simulink model "logging"  (R2021b)
settings: Solver=VariableStepAuto  StartTime=0.0  StopTime=10.0  RelTol=1e-3
undefined symbols (not defined in the file): DiscIntNeverNeededParam, magnitude, Newton, Raphson
libraries: simulink x4, slpidlib x1
settings Model: Creator=user  LastModifiedBy=cemery

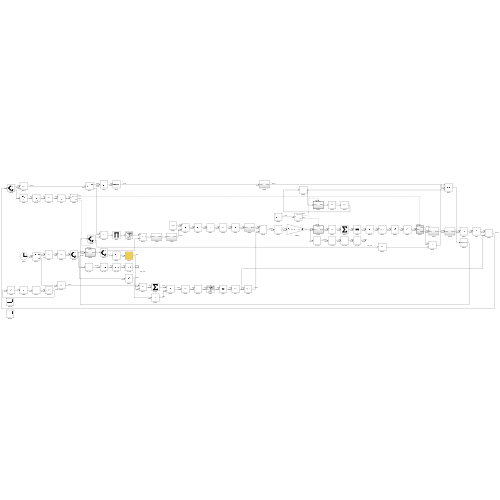
[thumbnail: Simulink's stored preview of the top-level diagram]
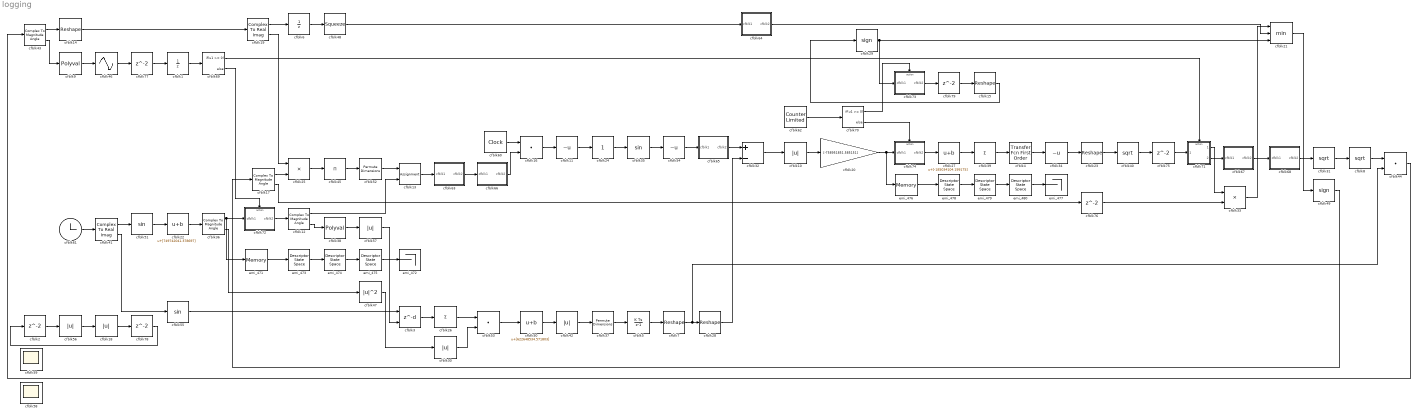
== system logging ==
  cfblk1 : UnitDelay  HasFrameUpgradeWarning=on
  cfblk{10,18,30,42,56..57} (6 alike) : Abs
  cfblk11 : UnaryMinus
  cfblk{12,17,36,43} (4 alike) : ComplexToMagnitudeAngle
  cfblk13 : Assignment  DiagnosticForDimensions=Warning  IndexOptions=Index vector (dialog)  Indices=1  OutputSizes=1
  cfblk{7,14..15,23,28} (5 alike) : Reshape
  cfblk16 : DotProduct  InputSameDT=on  OutDataTypeStr=Inherit: Inherit via internal rule
  cfblk19 : ComplexToRealImag
  cfblk{2,75..79} (6 alike) : Delay  SampleTime=1
  cfblk20 : Gain  Gain=[-758951851.585151]
  cfblk21 : MinMax  Inputs=3
  cfblk22 : Bias  Bias=[749742041.378697]
  cfblk24 : simulink/Math Operations/Slider Gain  gain=1  low=0  high=2
  cfblk25 : Product
  cfblk26 : Sum  Inputs=+
  cfblk27 : Bias  Bias=[-185034104.199175]
  cfblk29 : Signum
  cfblk3 : Delay  DelayLengthSource=Input port  SampleTime=1
      settings: InputPortMap=u0,p1
  cfblk31 : Sqrt  SaturateOnIntegerOverflow=on
  cfblk32 : Sum  Inputs=+-
  cfblk33 : Product
  cfblk34 : UnaryMinus
  cfblk35 : Trigonometry
  cfblk37 : PermuteDimensions
  cfblk38 : Polyval  Coefs=[ +2.081618890e-019, -1.441693666e-014, +4.719686976e-010, -8.536869453e-006, +1.621573104e-001, -8.087801117e+001 ]
  cfblk39 : Sum  Inputs=+
  cfblk4 : simulink/Discrete/Transfer Fcn First Order  PoleZ=0.95  ICPrevOutput=0.0  DoSatur=off
  cfblk40 : Sqrt  SaturateOnIntegerOverflow=on
  cfblk41 : ComplexToRealImag
  cfblk44 : DotProduct  InputSameDT=on  OutDataTypeStr=Inherit: Inherit via internal rule
  cfblk45 : Product  Inputs=*
  cfblk46 : Sin  TimeSource=Use external signal  SampleTime=0
  cfblk47 : Math  Operator=magnitude^2  SaturateOnIntegerOverflow=on
  cfblk48 : Squeeze
  cfblk49 : Signum
  cfblk5 : DiscreteIntegrator  ICPrevOutput=DiscIntNeverNeededParam  ICPrevScaledInput=DiscIntNeverNeededParam
  cfblk50 : Bias  Bias=[622648534.571803]
  cfblk51 : Trigonometry
  cfblk52 : PermuteDimensions
  cfblk53 : DotProduct  InputSameDT=on  OutDataTypeStr=Inherit: Inherit via internal rule
  cfblk54 : UnaryMinus
  cfblk55 : Trigonometry
  cfblk58 : Scope
      settings: Floating=on
  cfblk59 : Scope
      settings: Floating=on
  cfblk6 : UnitDelay  HasFrameUpgradeWarning=on
  cfblk60 : DigitalClock
  cfblk61 : Clock
  cfblk62 : simulink/Sources/Counter Limited  uplimit=[209.000000]  tsamp=-1
  cfblk63 : Subsystem
  cfblk64 : Subsystem
  cfblk65 : Subsystem
  cfblk66 : Subsystem
  cfblk67 : Subsystem
  cfblk68 : Subsystem
  cfblk69 : If  IfExpression=u1 >= 0  SampleTime=1
  cfblk70 : If  IfExpression=u1 >= 0  SampleTime=1
  cfblk71 : Subsystem  TreatAsAtomicUnit=on
  cfblk72 : Subsystem  TreatAsAtomicUnit=on
  cfblk73 : Subsystem  TreatAsAtomicUnit=on
  cfblk74 : Subsystem  TreatAsAtomicUnit=on
  cfblk8 : Sqrt  SaturateOnIntegerOverflow=on
  cfblk9 : Polyval  Coefs=[ +2.081618890e-019, -1.441693666e-014, +4.719686976e-010, -8.536869453e-006, +1.621573104e-001, -8.087801117e+001 ]
  emi_471 : Memory
  emi_472 : Terminator
  emi_{473..475,478..480} (6 alike) : DescriptorStateSpace
  emi_476 : Memory
  emi_477 : Terminator
  wires:
  cfblk47/1 -> cfblk30/1
  cfblk12/2 -> cfblk38/1
  emi_473/1 -> emi_474/1
  cfblk74/1(cfblk2) -> cfblk27/1
  cfblk18/1 -> cfblk78/1
  emi_480/1 -> emi_477/1
  emi_474/1 -> emi_475/1
  cfblk71/2(cfblk4) -> cfblk67/1(cfblk1)
  emi_479/1 -> emi_480/1
  cfblk68/1(cfblk2) -> cfblk31/1
  emi_478/1 -> emi_479/1
  cfblk78/1 -> cfblk2/1
  emi_476/1 -> emi_478/1
  cfblk77/1 -> cfblk1/1
  cfblk72/1(cfblk2) -> cfblk12/1
  cfblk66/1(cfblk2) -> cfblk16/2
  emi_475/1 -> emi_472/1
  emi_471/1 -> emi_473/1
  cfblk69/2 -> cfblk72/Action
  cfblk79/1 -> cfblk15/1
  cfblk62/1 -> cfblk70/1
  cfblk73/1(cfblk2) -> cfblk79/1
  cfblk19/2 -> cfblk25/1
  cfblk55/1 -> cfblk3/1
  cfblk76/1 -> cfblk33/2
  cfblk46/1 -> cfblk77/1
  cfblk54/1 -> cfblk65/1(cfblk1)
  cfblk17/2 -> cfblk76/1
  cfblk19/1 -> cfblk6/1
  cfblk75/1 -> cfblk71/1(cfblk1)
  cfblk21/1 -> cfblk49/1
  cfblk6/1 -> cfblk48/1
  cfblk70/2 -> cfblk74/Action
  cfblk40/1 -> cfblk75/1
  cfblk69/1 -> cfblk71/Action
  cfblk70/1 -> cfblk73/Action
  cfblk41/1 -> cfblk51/1
  cfblk67/1(cfblk2) -> cfblk68/1(cfblk1)
  cfblk28/1 -> cfblk32/2
  cfblk51/1 -> cfblk22/1
  cfblk61/1 -> cfblk41/1
  cfblk17/1 -> cfblk25/2
  cfblk52/1 -> cfblk13/1
  cfblk49/1 -> cfblk17/1
  cfblk10/1 -> cfblk20/1
  cfblk1/1 -> cfblk69/1
  cfblk3/1 -> cfblk26/1
  cfblk57/1 -> cfblk3/2
  cfblk2/1 -> cfblk56/1
  cfblk71/1(cfblk2) -> cfblk33/1
  cfblk50/1 -> cfblk42/1
  cfblk30/1 -> cfblk53/2
  cfblk14/1 -> cfblk19/1
  cfblk37/1 -> cfblk5/1
  cfblk41/2 -> cfblk55/1
  cfblk36/2 -> cfblk47/1
  cfblk64/1(cfblk2) -> cfblk21/2
  cfblk12/1 -> cfblk13/2
  cfblk53/1 -> cfblk50/1
  cfblk33/1 -> cfblk21/1
  cfblk16/1 -> cfblk11/1
  cfblk25/1 -> cfblk45/1
  cfblk60/1 -> cfblk16/1
  cfblk45/1 -> cfblk52/1
  cfblk15/1 -> cfblk29/1
  cfblk38/1 -> cfblk57/1
  cfblk9/1 -> cfblk46/1
  cfblk27/1 -> cfblk39/1
  cfblk32/1 -> cfblk10/1
  cfblk11/1 -> cfblk24/1
  cfblk22/1 -> cfblk36/1
  cfblk26/1 -> cfblk53/1
  cfblk44/1 -> cfblk43/1
  cfblk34/1 -> cfblk23/1
  cfblk8/1 -> cfblk44/1
  cfblk63/1(cfblk2) -> cfblk66/1(cfblk1)
  cfblk48/1 -> cfblk64/1(cfblk1)
  cfblk65/1(cfblk2) -> cfblk32/1
  cfblk31/1 -> cfblk8/1
  cfblk35/1 -> cfblk54/1
  cfblk4/1 -> cfblk34/1
  cfblk24/1 -> cfblk35/1
  cfblk43/2 -> cfblk9/1
  cfblk23/1 -> cfblk40/1
  cfblk13/1 -> cfblk63/1(cfblk1)
  cfblk42/1 -> cfblk37/1
  cfblk39/1 -> cfblk4/1
  cfblk43/1 -> cfblk14/1
  cfblk56/1 -> cfblk18/1
  cfblk5/1 -> cfblk7/1
  cfblk20/1 -> emi_476/1, cfblk74/1(cfblk1)
  cfblk36/1 -> emi_471/1, cfblk72/1(cfblk1)
  cfblk7/1 -> cfblk28/1, cfblk44/2
  cfblk29/1 -> cfblk73/1(cfblk1), cfblk21/3

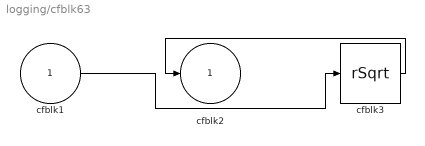
== system logging/cfblk63 ==
  cfblk1 : Inport
  cfblk3 : Sqrt  Operator=rSqrt  AlgorithmType=Newton-Raphson  SaturateOnIntegerOverflow=on
  cfblk2 : Outport
  wires:
  cfblk3/1 -> cfblk2/1
  cfblk1/1 -> cfblk3/1

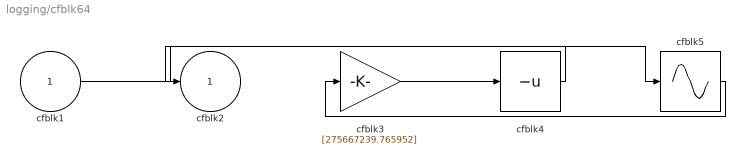
== system logging/cfblk64 ==
  cfblk1 : Inport
  cfblk3 : Gain  Gain=[275667239.765952]
  cfblk4 : UnaryMinus
  cfblk5 : Sin  TimeSource=Use external signal  SampleTime=0
  cfblk2 : Outport
  wires:
  cfblk1/1 -> cfblk5/1
  cfblk3/1 -> cfblk4/1
  cfblk5/1 -> cfblk3/1
  cfblk4/1 -> cfblk2/1

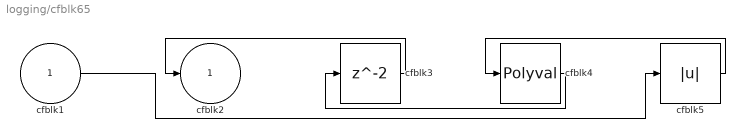
== system logging/cfblk65 ==
  cfblk1 : Inport
  cfblk3 : Delay  SampleTime=1
  cfblk4 : Polyval  Coefs=[ +2.081618890e-019, -1.441693666e-014, +4.719686976e-010, -8.536869453e-006, +1.621573104e-001, -8.087801117e+001 ]
  cfblk5 : Abs
  cfblk2 : Outport
  wires:
  cfblk3/1 -> cfblk2/1
  cfblk5/1 -> cfblk4/1
  cfblk4/1 -> cfblk3/1
  cfblk1/1 -> cfblk5/1

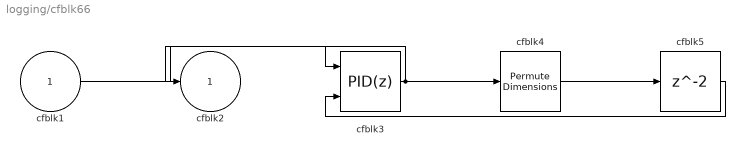
== system logging/cfblk66 ==
  cfblk1 : Inport
  cfblk3 : slpidlib/PID Controller (2DOF)  Controller=PID  Form=Parallel  TimeDomain=Discrete-time  UseExternalTs=off  SampleTime=1  IntegratorMethod=Forward Euler  FilterMethod=Forward Euler  ControllerParametersSource=internal  P=1  I=1  D=0  UseFilter=on  N=100  b=1  c=1  TunerSelectOption=Transfer Function Based (PID Tuner App)  InitialConditionSource=internal  InitialConditionForIntegrator=0  InitialConditionForFilter=0  DifferentiatorICPrevScaledInput=0  ExternalReset=none  TrackingMode=off  Kt=1  LimitOutput=off  SatLimitsSource=internal  UpperSaturationLimit=inf  LowerSaturationLimit=-inf  LinearizeAsGain=off  AntiWindupMode=none  Kb=1  POutMin=[]  POutMax=[]  IOutMin=[]  IOutMax=[]  DOutMin=[]  DOutMax=[]  NOutMin=[]  NOutMax=[]  bOutMin=[]  bOutMax=[]  cOutMin=[]  cOutMax=[]  SumOutMin=[]  SumOutMax=[]  SaturationOutMin=[]  SaturationOutMax=[]  PParamMin=[]  PParamMax=[]  IParamMin=[]  IParamMax=[]  DParamMin=[]  DParamMax=[]  NParamMin=[]  NParamMax=[]  bParamMin=[]  bParamMax=[]  cParamMin=[]  cParamMax=[]  KbParamMin=[]  KbParamMax=[]  KtParamMin=[]  KtParamMax=[]  KbOutMin=[]  KbOutMax=[]  KtOutMin=[]  KtOutMax=[]  IntegratorOutMin=[]  IntegratorOutMax=[]  FilterOutMin=[]  FilterOutMax=[]  SumI1OutMin=[]  SumI1OutMax=[]  SumI2OutMin=[]  SumI2OutMax=[]  SumI3OutMin=[]  SumI3OutMax=[]  SumI4OutMin=[]  SumI4OutMax=[]  SumDOutMin=[]  SumDOutMax=[]  Sum1OutMin=[]  Sum1OutMax=[]  Sum2OutMin=[]  Sum2OutMax=[]  Sum3OutMin=[]  Sum3OutMax=[]  DifferentiatorOutMin=[]  DifferentiatorOutMax=[]  FilterDiffOutCoefMin=[]  FilterDiffOutCoefMax=[]  ReciprocalOutMin=[]  ReciprocalOutMax=[]  SumDenOutMin=[]  SumDenOutMax=[]  SumNumOutMin=[]  SumNumOutMax=[]  DivideOutMin=[]  DivideOutMax=[]  UdiffTsProdOutMin=[]  UdiffTsProdOutMax=[]  NTsProdOutMin=[]  NTsProdOutMax=[]  UintegralTsProdOutMin=[]  UintegralTsProdOutMax=[]  UngainTsProdOutMin=[]  UngainTsProdOutMax=[]  IntegratorContinuousStateAttributes=''  IntegratorStateMustResolveToSignalObject=off  IntegratorRTWStateStorageClass=Auto  FilterContinuousStateAttributes=''  FilterStateMustResolveToSignalObject=off  FilterRTWStateStorageClass=Auto  ParallelPVariant=InternalParameters  IdealPVariant=Disabled  IVariant=InternalParameters  DVariant=InternalParameters  bVariant=InternalParameters  cVariant=InternalParameters  IntegratorVariant=Discrete  SatVariant=Disabled  AWVariant=Passthrough  PCopyVariant=Disabled  TRVariant=Disabled  FdbkBlocksVariant=Forward  IdealPFdbkVariant=Disabled  SatFdbkVariant=Disabled  DerivativeFilterVariant=ForwardEulerFilter  NVariant=InternalParameters  NCopyVariant=Disabled  FilterICVariant=InternalICsFilter  IntegratorICVariant=InternalICs  ExternalResetVariant=Disabled  TRSumVariant=Passthrough  SumFdbkVariant=Disabled  SumVariant=Sum_PID  TsampFilterVariant=InternalTs  TsampNgainVariant=Passthrough  TsampIntegralVariant=Passthrough  ExternalSaturationOutDataTypeStr=Inherit: Same as second input
      settings: SourceProductBaseCode=SL
  cfblk4 : PermuteDimensions
  cfblk5 : Delay  SampleTime=1
  cfblk2 : Outport
  wires:
  cfblk3/1 -> cfblk4/1, cfblk2/1
  cfblk1/1 -> cfblk3/1
  cfblk4/1 -> cfblk5/1
  cfblk5/1 -> cfblk3/2

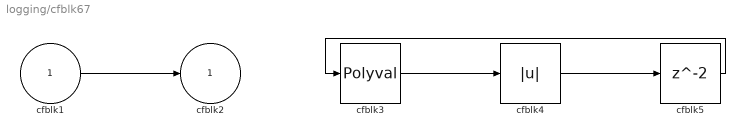
== system logging/cfblk67 ==
  cfblk1 : Inport
  cfblk3 : Polyval  Coefs=[ +2.081618890e-019, -1.441693666e-014, +4.719686976e-010, -8.536869453e-006, +1.621573104e-001, -8.087801117e+001 ]
  cfblk4 : Abs
  cfblk5 : Delay  SampleTime=1
  cfblk2 : Outport
  wires:
  cfblk1/1 -> cfblk2/1
  cfblk3/1 -> cfblk4/1
  cfblk4/1 -> cfblk5/1
  cfblk5/1 -> cfblk3/1

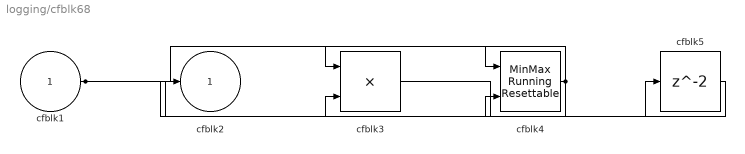
== system logging/cfblk68 ==
  cfblk1 : Inport
  cfblk3 : Product
  cfblk4 : simulink/Math Operations/MinMax Running Resettable  Function=min  vinit=0.0
  cfblk5 : Delay  SampleTime=1
  cfblk2 : Outport
  wires:
  cfblk1/1 -> cfblk4/1, cfblk3/2
  cfblk4/1 -> cfblk2/1, cfblk3/1
  cfblk3/1 -> cfblk5/1
  cfblk5/1 -> cfblk4/2

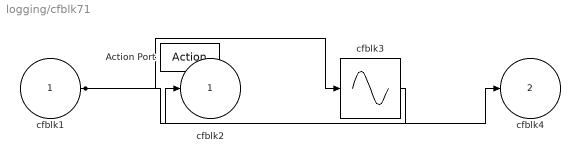
== system logging/cfblk71 ==
  cfblk1 : Inport
  Action Port : ActionPort  ActionPortLabel=if(u1 >= 0)
  cfblk3 : Sin  TimeSource=Use external signal  SampleTime=0
  cfblk2 : Outport
  cfblk4 : Outport  Port=2
  wires:
  cfblk3/1 -> cfblk2/1
  cfblk1/1 -> cfblk3/1, cfblk4/1

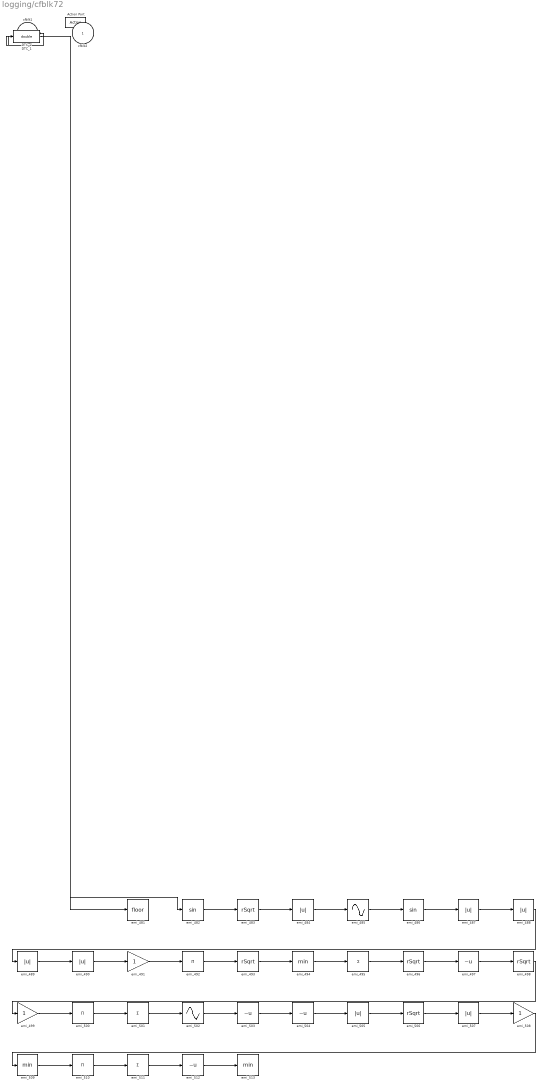
== system logging/cfblk72 ==
  cfblk1 : Inport
  Action Port : ActionPort  ActionPortLabel=else
  DTC_1 : DataTypeConversion  OutDataTypeStr=double
  DTC_2 : DataTypeConversion  OutDataTypeStr=double
  emi_481 : Rounding
  emi_482 : Trigonometry
  emi_{483,493,496,498,506} (5 alike) : Sqrt  Operator=rSqrt  SaturateOnIntegerOverflow=on
  emi_{484,487..490,505,507} (7 alike) : Abs
  emi_485 : Sin  TimeSource=Use external signal  SampleTime=0
  emi_486 : Trigonometry
  emi_491 : Gain
  emi_492 : Product  Inputs=*
  emi_494 : MinMax
  emi_495 : Sum  Inputs=+
  emi_{497,503..504,512} (4 alike) : UnaryMinus
  emi_499 : Gain
  emi_500 : Product  Inputs=*
  emi_501 : Sum  Inputs=+
  emi_502 : Sin  TimeSource=Use external signal  SampleTime=0
  emi_508 : Gain
  emi_509 : MinMax
  emi_510 : Product  Inputs=*
  emi_511 : Sum  Inputs=+
  emi_513 : MinMax
  cfblk2 : Outport
  wires:
  cfblk1/1 -> DTC_1/1, DTC_2/1
  DTC_1/1 -> emi_481/1
  DTC_2/1 -> emi_482/1
  emi_482/1 -> emi_483/1
  emi_483/1 -> emi_484/1
  emi_484/1 -> emi_485/1
  emi_485/1 -> emi_486/1
  emi_486/1 -> emi_487/1
  emi_487/1 -> emi_488/1
  emi_488/1 -> emi_489/1
  emi_489/1 -> emi_490/1
  emi_490/1 -> emi_491/1
  emi_491/1 -> emi_492/1
  emi_492/1 -> emi_493/1
  emi_493/1 -> emi_494/1
  emi_494/1 -> emi_495/1
  emi_495/1 -> emi_496/1
  emi_496/1 -> emi_497/1
  emi_497/1 -> emi_498/1
  emi_498/1 -> emi_499/1
  emi_499/1 -> emi_500/1
  emi_500/1 -> emi_501/1
  emi_501/1 -> emi_502/1
  emi_502/1 -> emi_503/1
  emi_503/1 -> emi_504/1
  emi_504/1 -> emi_505/1
  emi_505/1 -> emi_506/1
  emi_506/1 -> emi_507/1
  emi_507/1 -> emi_508/1
  emi_508/1 -> emi_509/1
  emi_509/1 -> emi_510/1
  emi_510/1 -> emi_511/1
  emi_511/1 -> emi_512/1
  emi_512/1 -> emi_513/1

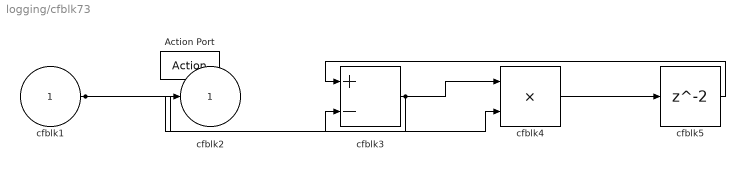
== system logging/cfblk73 ==
  cfblk1 : Inport
  Action Port : ActionPort  ActionPortLabel=if(u1 >= 0)
  cfblk3 : Sum  Inputs=+-
  cfblk4 : Product  Inputs=**
  cfblk5 : Delay
  cfblk2 : Outport
  wires:
  cfblk3/1 -> cfblk4/1, cfblk2/1
  cfblk1/1 -> cfblk3/2, cfblk4/2
  cfblk4/1 -> cfblk5/1
  cfblk5/1 -> cfblk3/1

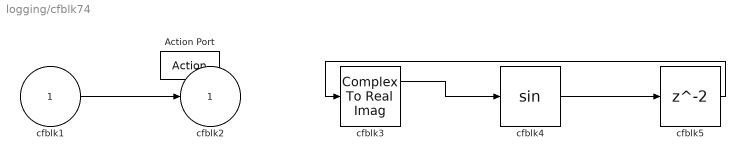
== system logging/cfblk74 ==
  cfblk1 : Inport
  Action Port : ActionPort  ActionPortLabel=else
  cfblk3 : ComplexToRealImag
  cfblk4 : Trigonometry
  cfblk5 : Delay
  cfblk2 : Outport
  wires:
  cfblk1/1 -> cfblk2/1
  cfblk3/1 -> cfblk4/1
  cfblk4/1 -> cfblk5/1
  cfblk5/1 -> cfblk3/1
